simulink model "asbCubeSatVisualization"  (R2022a)
settings: configuration reference "CubeSatConfigSet" (kept outside this file)
undefined symbols (not defined in the file): altitude
libraries: aerolibutil x7, aerolibconvert2 x3, aerolibobsolete x1, aerolibattitudesys x1, simulink x1, vrlib x1
settings Model: DataDictionary=asbCubeSatArchInterfaceData.sldd  Creator=The MathWorks, Inc.  LastModifiedBy=4jack
settings ConfigSetRef: SourceName=CubeSatConfigSet

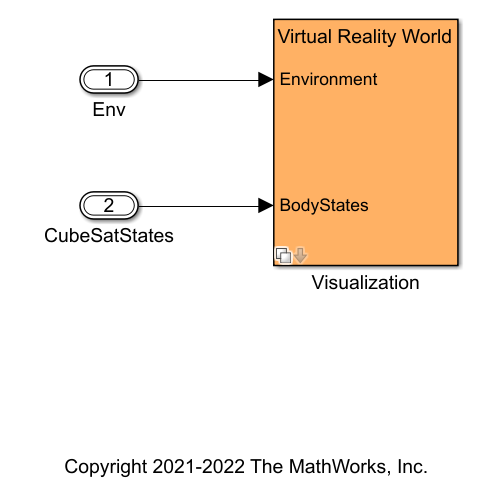
[thumbnail: Simulink's stored preview of the top-level diagram]
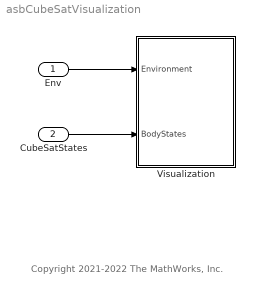
== system asbCubeSatVisualization ==
  note: Copyright 2021-2022 The MathWorks, Inc.
  Env : Inport  OutDataTypeStr=Bus: EnvBus
  CubeSatStates : Inport  Port=2  OutDataTypeStr=Bus: StatesOutBus
  Visualization : Subsystem  Variant=on  mask(Set Animation Properties){visSampleTime=5, cubesatSize=2e5, showAntenna=on, antennaHeight=-1*(altitude - 6317000), antennaHalfAngle=25}
      mask prompts: visSampleTime "spacecraft:cubesat:AnimSampleTime"; cubesatSize "spacecraft:cubesat:MdlSize"; showAntenna "spacecraft:cubesat:ShowCone"; antennaHeight "spacecraft:cubesat:ConeHeight"; antennaHalfAngle "spacecraft:cubesat:ConeAngle"
      mask help: spacecraft:cubesat:VisBlockDesc
      mask Callback showAntenna:
      | if builtin('license','test','Virtual_Reality_Toolbox')
      | 
      |     enable = get_param(gcb,'MaskEnables');
      |     if strcmp(get_param(gcb, 'showAntenna'), 'off')
      |         enable(4:5) = {'off'};
      |     else
      |         enable(4:5) = {'on'};
      |     end
      |     set_param(gcb,'MaskEnables', enable);
      |     clear enable
      | end
      mask DialogControl vrOpenBtn Prompt: spacecraft:cubesat:AnimOpenBtn
      mask DialogControl vrOpenBtn Callback:
      | if builtin('license','checkout','Virtual_Reality_Toolbox')
      |     vrmfunc('FnOpen',getSimulinkBlockHandle([gcb '/Virtual Reality World/VR Sink']));
      | end
      mask DialogControl visSampleTime Prompt: Animation refresh rate:
      mask DialogControl visSampleTime Tooltip: spacecraft:cubesat:AnimSampleTimeTT
      mask DialogControl cubesatSize Prompt: CubeSat display size [m]:
      mask DialogControl cubesatSize Tooltip: spacecraft:cubesat:MdlSizeTT
      mask DialogControl Container3 Prompt: spacecraft:cubesat:AntennaPropArea
      mask DialogControl showAntenna Prompt: Show antenna cone in animation
      mask DialogControl showAntenna Tooltip: spacecraft:cubesat:ShowConeTT
      mask DialogControl antennaHeight Prompt: Antenna cone height [m]:
      mask DialogControl antennaHeight Tooltip: spacecraft:cubesat:ConeHeightTT
      mask DialogControl antennaHalfAngle Prompt: Antenna cone half angle [deg]:
      mask DialogControl antennaHalfAngle Tooltip: spacecraft:cubesat:ConeAngleTT
  wires:
  CubeSatStates/1 -> Visualization/2(BodyStates)
  Env/1 -> Visualization/1(Environment)

== system asbCubeSatVisualization/Visualization ==
  Environment : Inport
  BodyStates : Inport  RequirementInfo={} %GIDa_10e629f3_1d72_465b_94cc_14990dd9aecc  Port=2
  No Visualization : Subsystem  VariantControl=visOff
  Virtual Reality World : Subsystem  VariantControl=visSL3D

== system asbCubeSatVisualization/Visualization/No Visualization ==
  BodyStates : Inport
  Environment : Inport  Port=2
  Terminator2 : Terminator
      settings: RequirementInfo={} %GIDa_0fc65eef_4c11_4565_975b_7fa0252905f4
  Terminator3 : Terminator
      settings: RequirementInfo={} %GIDa_377e63f1_3103_416f_a52c_127c2ec39819
  wires:
  BodyStates/1 -> Terminator3/1
  Environment/1 -> Terminator2/1

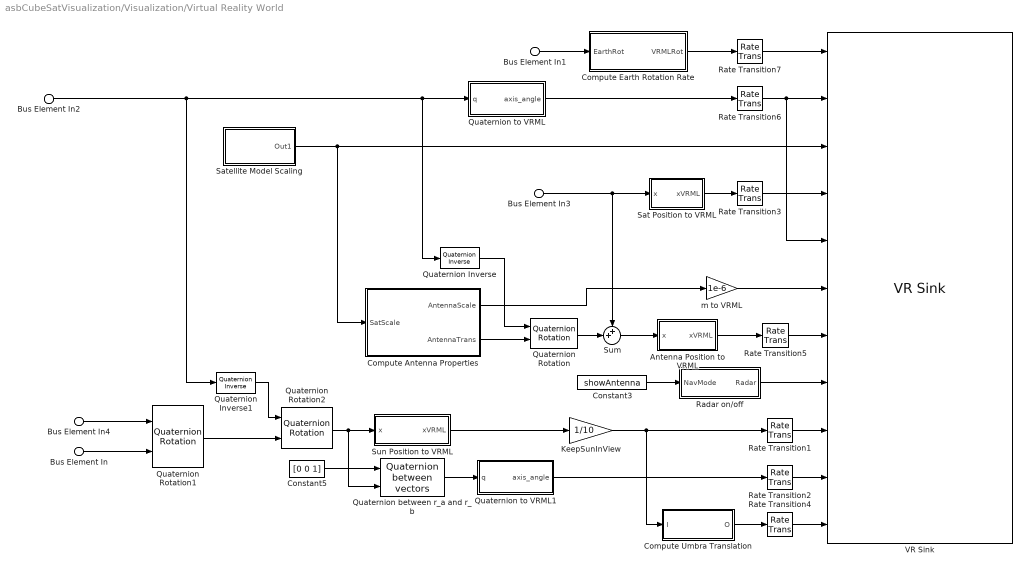
== system asbCubeSatVisualization/Visualization/Virtual Reality World ==
  Bus Element In3 : Inport  PortName=BodyStates  Element=X_ecef
  Bus Element In2 : Inport  PortName=BodyStates  Element=q_ecef2b
  Bus Element In4 : Inport  PortName=BodyStates  Element=q_eci2b
  Bus Element In : Inport  Port=2  PortName=Environment  Element=x_sun_eci
  Bus Element In1 : Inport  Port=2  PortName=Environment  Element=earthAngRate
  Antenna Position to VRML : Subsystem
  Compute Antenna Properties : Subsystem
  Compute Earth Rotation Rate : Subsystem
  Compute Umbra Translation : Subsystem
  Constant3 : Constant  Value=showAntenna
  Constant5 : Constant  Value=[0 0 1]
  KeepSunInView : Gain  Gain=1/10
  Quaternion Inverse : aerolibutil/Quaternion Inverse
  Quaternion Inverse1 : aerolibutil/Quaternion Inverse
  Quaternion Rotation : aerolibutil/Quaternion Rotation
  Quaternion Rotation1 : aerolibutil/Quaternion Rotation
  Quaternion Rotation2 : aerolibutil/Quaternion Rotation
  Quaternion between r_a and r_b : aerolibattitudesys/Quaternion between vectors
      settings: SourceProductBaseCode=AE
  Quaternion to VRML : Subsystem
  Quaternion to VRML1 : Subsystem
  Radar on/off : Subsystem
  Rate Transition{1..7} (7 alike) : RateTransition
  Sat Position to VRML : Subsystem
  Satellite Model Scaling : Subsystem
  Sum : Sum  Inputs=++|
  Sun Position to VRML : Subsystem
  VR Sink : vrlib/VR Sink  InstantiateOnLoad=on  SampleTime=visSampleTime  ViewEnable=on  RemoteChange=off  RemoteView=off  FieldsWritten=Earth.rotation.4.1.1.double#Satellite.rotation.4.1.1.double#Satellite.scale.3.1.1.double#Satellite.translation.3.1.1.double#AntennaCone.rotation.4.1.1.double#AntennaCone.scale.3.1.1.double#AntennaCone.translation.3.1.1.double#AntennaMaterial.transparency.1.1.1.double#Sun.translation.3.1.1.double#Umbra.rotation.4.1.1.double#Umbra.translation.3.1.1.double  WorldFileName=cubesatAnim.wrl  WorldDescription=CubeSat Orbit Animation  AutoView=on  VideoDimensions=[]  AllowVariableSize=off  FigureProperties="{'Position', 'Name', 'Viewpoint', 'CameraBound', 'CameraDirection', 'CameraPosition', 'CameraUpVector', 'ZoomFactor', 'Antialiasing', 'Headlight', 'Lighting', 'NavPanel', 'Sound', 'StatusBar', 'Stereo3D', 'Stereo3DCameraOffset', 'Stereo3DHIT', 'ToolBar', 'Textures', 'Transparency', 'Triad', 'Wireframe', 'NavZones', 'NavMode', 'NavSpeed', 'CaptureFileFormat', 'CaptureFileName', 'Record2DCompressMethod', 'Record2DCompressQuality', 'Record2D', 'Record2DFileName', 'Record2DFPS'; [5.0000000000000000e+00   9.2000000000000000e+01   5.7600000000000000e+02   3.5000000000000000e+02], 'CubeSat Orbit Animation', 'NorthPole', 'on', [0.0000000000000000e+00   0.0000000000000000e+00  -1.0000000000000000e+00], [0.0000000000000000e+00   0.0000000000000000e+00   0.0000000000000000e+00], [0.0000000000000000e+00   1.0000000000000000e+00   0.0000000000000000e+00], [1.0000000000000000e+00], 'on', 'on', 'on', 'halfbar', 'on', 'on', 'off', [1.0000000149011612e-01], [0.0000000000000000e+00], 'on', 'on', 'on', 'none', 'off', 'off', 'examine', 'normal', 'tif', '%f_anim_%n.tif', 'auto', [7.5000000000000000e+01], 'off', '%f_anim_%n.avi', 'auto'; [5.0000000000000000e+00   9.2000000000000000e+01   5.7600000000000000e+02   3.5000000000000000e+02], 'CubeSat Orbit Animation', 'NorthPole', 'on', [0.0000000000000000e+00   0.0000000000000000e+00  -1.0000000000000000e+00], [0.0000000000000000e+00   0.0000000000000000e+00   0.0000000000000000e+00], [0.0000000000000000e+00   1.0000000000000000e+00   0.0000000000000000e+00], [1.0000000000000000e+00], 'on', 'on', 'on', 'halfbar', 'on', 'on', 'off', [1.0000000149011612e-01], [0.0000000000000000e+00], 'on', 'on', 'on', 'none', 'off', 'off', 'examine', 'normal', 'tif', '%f_anim_%n.tif', 'auto', [7.5000000000000000e+01], 'off', '%f_anim_%n.avi', 'auto'}"
  m to VRML : Gain  Gain=1e-6
  wires:
  Rate Transition6/1 -> VR Sink/2, VR Sink/5
  Quaternion to VRML/1(axis_angle) -> Rate Transition6/1
  Rate Transition5/1 -> VR Sink/7
  Rate Transition3/1 -> VR Sink/4
  Rate Transition7/1 -> VR Sink/1
  Bus Element In1/1 -> Compute Earth Rotation Rate/1(EarthRot)
  Rate Transition2/1 -> VR Sink/10
  Rate Transition1/1 -> VR Sink/9
  Rate Transition4/1 -> VR Sink/11
  Bus Element In/1 -> Quaternion Rotation1/2
  Bus Element In4/1 -> Quaternion Rotation1/1
  Compute Antenna Properties/2(AntennaTrans) -> Quaternion Rotation/2
  Compute Antenna Properties/1(AntennaScale) -> m to VRML/1
  Satellite Model Scaling/1(Out1) -> Compute Antenna Properties/1(SatScale), VR Sink/3
  Compute Umbra Translation/1(O) -> Rate Transition4/1
  KeepSunInView/1 -> Rate Transition1/1, Compute Umbra Translation/1(I)
  Quaternion to VRML1/1(axis_angle) -> Rate Transition2/1
  Radar on/off/1(Radar) -> VR Sink/8
  Sat Position to VRML/1(xVRML) -> Rate Transition3/1
  Compute Earth Rotation Rate/1(VRMLRot) -> Rate Transition7/1
  Antenna Position to VRML/1(xVRML) -> Rate Transition5/1
  m to VRML/1 -> VR Sink/6
  Constant5/1 -> Quaternion between r_a and r_b/1
  Quaternion between r_a and r_b/1 -> Quaternion to VRML1/1(q)
  Sun Position to VRML/1(xVRML) -> KeepSunInView/1
  Quaternion Inverse1/1 -> Quaternion Rotation2/1
  Quaternion Rotation1/1 -> Quaternion Rotation2/2
  Quaternion Rotation2/1 -> Quaternion between r_a and r_b/2, Sun Position to VRML/1(x)
  Quaternion Rotation/1 -> Sum/2
  Sum/1 -> Antenna Position to VRML/1(x)
  Quaternion Inverse/1 -> Quaternion Rotation/1
  Bus Element In3/1 -> Sum/1, Sat Position to VRML/1(x)
  Constant3/1 -> Radar on/off/1(NavMode)
  Bus Element In2/1 -> Quaternion Inverse1/1, Quaternion Inverse/1, Quaternion to VRML/1(q)

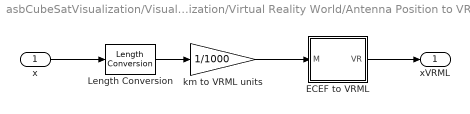
== system asbCubeSatVisualization/Visualization/Virtual Reality World/Antenna Position to VRML ==
  x : Inport
  ECEF to VRML : Subsystem
  Length Conversion : aerolibconvert2/Length Conversion  IU=m  OU=km
  km to VRML units : Gain  Gain=1/1000
  xVRML : Outport  VectorParamsAs1DForOutWhenUnconnected=off
  wires:
  ECEF to VRML/1(VR) -> xVRML/1
  x/1 -> Length Conversion/1
  km to VRML units/1 -> ECEF to VRML/1(M)
  Length Conversion/1 -> km to VRML units/1

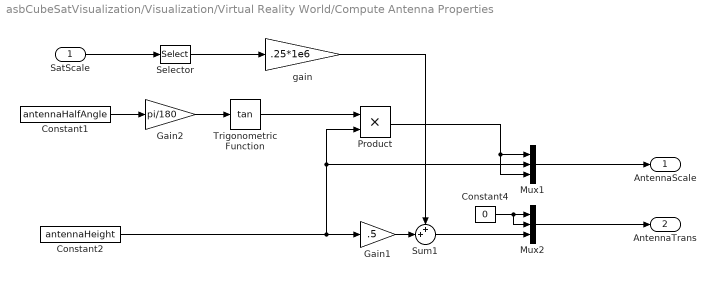
== system asbCubeSatVisualization/Visualization/Virtual Reality World/Compute Antenna Properties ==
  SatScale : Inport
  Constant1 : Constant  Value=antennaHalfAngle
  Constant2 : Constant  Value=antennaHeight
  Constant4 : Constant  Value=0
  Gain1 : Gain  Gain=.5
  Gain2 : Gain  Gain=pi/180
  Mux1 : Mux  Inputs=3
  Mux2 : Mux  Inputs=3
  Product : Product
  Selector : Selector  InputPortWidth=3  IndexOptions=Index vector (dialog)  Indices=1  OutputSizes=1
  Sum1 : Sum  Inputs=++|
  Trigonometric Function : Trigonometry  Operator=tan
  gain : Gain  Gain=.25*1e6
  AntennaScale : Outport  VectorParamsAs1DForOutWhenUnconnected=off
  AntennaTrans : Outport  Port=2  VectorParamsAs1DForOutWhenUnconnected=off
  wires:
  Selector/1 -> gain/1
  SatScale/1 -> Selector/1
  Mux1/1 -> AntennaScale/1
  Mux2/1 -> AntennaTrans/1
  Trigonometric Function/1 -> Product/1
  Gain1/1 -> Sum1/2
  Product/1 -> Mux1/1, Mux1/3
  Constant1/1 -> Gain2/1
  gain/1 -> Sum1/1
  Constant2/1 -> Product/2, Mux1/2, Gain1/1
  Sum1/1 -> Mux2/3
  Constant4/1 -> Mux2/2, Mux2/1
  Gain2/1 -> Trigonometric Function/1

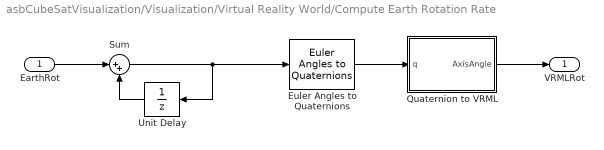
== system asbCubeSatVisualization/Visualization/Virtual Reality World/Compute Earth Rotation Rate ==
  EarthRot : Inport
  Euler Angles to Quaternions : aerolibobsolete/Euler Angles to Quaternions
      settings: SourceProductBaseCode=AE
  Quaternion to VRML : Subsystem
  Sum : Sum  Inputs=|++
  Unit Delay : UnitDelay  SampleTime=-1  HasFrameUpgradeWarning=on
  VRMLRot : Outport  VectorParamsAs1DForOutWhenUnconnected=off
  wires:
  Quaternion to VRML/1(AxisAngle) -> VRMLRot/1
  Euler Angles to Quaternions/1 -> Quaternion to VRML/1(q)
  Sum/1 -> Euler Angles to Quaternions/1, Unit Delay/1
  Unit Delay/1 -> Sum/2
  EarthRot/1 -> Sum/1

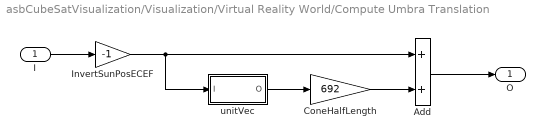
== system asbCubeSatVisualization/Visualization/Virtual Reality World/Compute Umbra Translation ==
  I : Inport
  Add : Sum
  ConeHalfLength : Gain  Gain=692
  InvertSunPosECEF : Gain  Gain=-1
  unitVec : Subsystem
  O : Outport  VectorParamsAs1DForOutWhenUnconnected=off
  wires:
  unitVec/1(O) -> ConeHalfLength/1
  InvertSunPosECEF/1 -> Add/1, unitVec/1(I)
  Add/1 -> O/1
  I/1 -> InvertSunPosECEF/1
  ConeHalfLength/1 -> Add/2

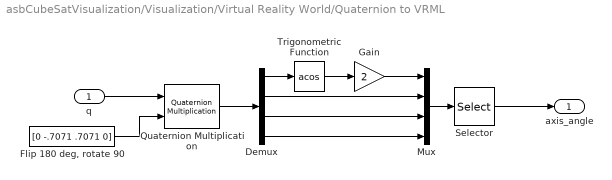
== system asbCubeSatVisualization/Visualization/Virtual Reality World/Quaternion to VRML ==
  q : Inport
  Demux : Demux
  "Flip 180 deg, rotate 90" : Constant  Value=[0 -.7071 .7071 0]
  Gain : Gain  Gain=2
  Mux : Mux
  Quaternion Multiplication : aerolibutil/Quaternion Multiplication
  Selector : Selector  InputPortWidth=4  IndexOptions=Index vector (dialog)  Indices=[3 4 2 1]  OutputSizes=1
  Trigonometric Function : Trigonometry  Operator=acos
  axis_angle : Outport  VectorParamsAs1DForOutWhenUnconnected=off
  wires:
  Quaternion Multiplication/1 -> Demux/1
  "Flip 180 deg, rotate 90"/1 -> Quaternion Multiplication/2
  Demux/1 -> Trigonometric Function/1
  Trigonometric Function/1 -> Gain/1
  Mux/1 -> Selector/1
  q/1 -> Quaternion Multiplication/1
  Selector/1 -> axis_angle/1
  Gain/1 -> Mux/1
  Demux/2 -> Mux/2
  Demux/3 -> Mux/3
  Demux/4 -> Mux/4

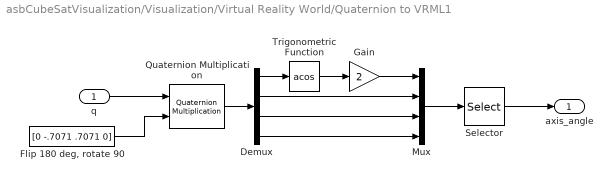
== system asbCubeSatVisualization/Visualization/Virtual Reality World/Quaternion to VRML1 ==
  q : Inport
  Demux : Demux
  "Flip 180 deg, rotate 90" : Constant  Value=[0 -.7071 .7071 0]
  Gain : Gain  Gain=2
  Mux : Mux
  Quaternion Multiplication : aerolibutil/Quaternion Multiplication
  Selector : Selector  InputPortWidth=4  IndexOptions=Index vector (dialog)  Indices=[3 4 2 1]  OutputSizes=1
  Trigonometric Function : Trigonometry  Operator=acos
  axis_angle : Outport  VectorParamsAs1DForOutWhenUnconnected=off
  wires:
  Quaternion Multiplication/1 -> Demux/1
  q/1 -> Quaternion Multiplication/1
  "Flip 180 deg, rotate 90"/1 -> Quaternion Multiplication/2
  Demux/1 -> Trigonometric Function/1
  Trigonometric Function/1 -> Gain/1
  Mux/1 -> Selector/1
  Selector/1 -> axis_angle/1
  Gain/1 -> Mux/1
  Demux/2 -> Mux/2
  Demux/3 -> Mux/3
  Demux/4 -> Mux/4

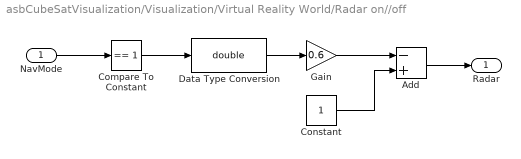
== system asbCubeSatVisualization/Visualization/Virtual Reality World/Radar on//off ==
  NavMode : Inport
  Add : Sum  Inputs=-+
  Compare To Constant : simulink/Logic and Bit Operations/Compare To Constant  relop===  const=1  OutDataTypeStr=boolean  ZeroCross=off
  Constant : Constant
  Data Type Conversion : DataTypeConversion  OutDataTypeStr=double  SaturateOnIntegerOverflow=off  RndMeth=Floor
  Gain : Gain  Gain=0.6
  Radar : Outport  VectorParamsAs1DForOutWhenUnconnected=off
  wires:
  Add/1 -> Radar/1
  Constant/1 -> Add/2
  Gain/1 -> Add/1
  Data Type Conversion/1 -> Gain/1
  Compare To Constant/1 -> Data Type Conversion/1
  NavMode/1 -> Compare To Constant/1

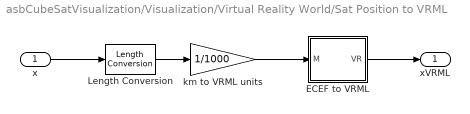
== system asbCubeSatVisualization/Visualization/Virtual Reality World/Sat Position to VRML ==
  x : Inport
  ECEF to VRML : Subsystem
  Length Conversion : aerolibconvert2/Length Conversion  IU=m  OU=km
  km to VRML units : Gain  Gain=1/1000
  xVRML : Outport  VectorParamsAs1DForOutWhenUnconnected=off
  wires:
  Length Conversion/1 -> km to VRML units/1
  km to VRML units/1 -> ECEF to VRML/1(M)
  x/1 -> Length Conversion/1
  ECEF to VRML/1(VR) -> xVRML/1

== system asbCubeSatVisualization/Visualization/Virtual Reality World/Satellite Model Scaling ==
  Constant : Constant  Value=cubesatSize
  Mux : Mux  Inputs=3
  ScaleModelToVRML : Gain  Gain=1/.3e6
  Out1 : Outport  VectorParamsAs1DForOutWhenUnconnected=off
  wires:
  Mux/1 -> Out1/1
  Constant/1 -> ScaleModelToVRML/1
  ScaleModelToVRML/1 -> Mux/2, Mux/1, Mux/3

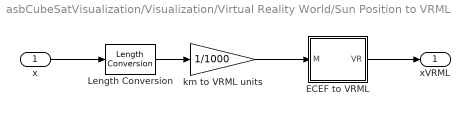
== system asbCubeSatVisualization/Visualization/Virtual Reality World/Sun Position to VRML ==
  x : Inport
  ECEF to VRML : Subsystem
  Length Conversion : aerolibconvert2/Length Conversion  IU=m  OU=km
  km to VRML units : Gain  Gain=1/1000
  xVRML : Outport  VectorParamsAs1DForOutWhenUnconnected=off
  wires:
  Length Conversion/1 -> km to VRML units/1
  km to VRML units/1 -> ECEF to VRML/1(M)
  x/1 -> Length Conversion/1
  ECEF to VRML/1(VR) -> xVRML/1

== system asbCubeSatVisualization/Visualization/Virtual Reality World/Antenna Position to VRML/ECEF to VRML ==
  M : Inport  PortDimensions=3
  Selector : Selector  InputPortWidth=3  IndexOptions=Index vector (dialog)  Indices=[2 3 1]  OutputSizes=1
  VR : Outport  PortDimensions=3  VectorParamsAs1DForOutWhenUnconnected=off
  wires:
  Selector/1 -> VR/1
  M/1 -> Selector/1

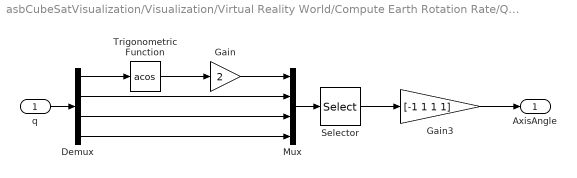
== system asbCubeSatVisualization/Visualization/Virtual Reality World/Compute Earth Rotation Rate/Quaternion to VRML ==
  q : Inport
  Demux : Demux
  Gain : Gain  Gain=2
  Gain3 : Gain  Gain=[-1 1 1 1]
  Mux : Mux
  Selector : Selector  InputPortWidth=4  IndexOptions=Index vector (dialog)  Indices=[2 4 3 1]  OutputSizes=1
  Trigonometric Function : Trigonometry  Operator=acos
  AxisAngle : Outport  VectorParamsAs1DForOutWhenUnconnected=off
  wires:
  Demux/1 -> Trigonometric Function/1
  Trigonometric Function/1 -> Gain/1
  Mux/1 -> Selector/1
  q/1 -> Demux/1
  Gain3/1 -> AxisAngle/1
  Selector/1 -> Gain3/1
  Gain/1 -> Mux/1
  Demux/2 -> Mux/2
  Demux/3 -> Mux/3
  Demux/4 -> Mux/4

== system asbCubeSatVisualization/Visualization/Virtual Reality World/Compute Umbra Translation/unitVec ==
  I : Inport
  Divide : Product  Inputs=*/
  Dot Product : DotProduct  OutDataTypeStr=Inherit: Inherit via internal rule
  Sqrt : Sqrt
  O : Outport  VectorParamsAs1DForOutWhenUnconnected=off
  wires:
  Sqrt/1 -> Divide/2
  Divide/1 -> O/1
  I/1 -> Dot Product/2, Dot Product/1, Divide/1
  Dot Product/1 -> Sqrt/1

== system asbCubeSatVisualization/Visualization/Virtual Reality World/Sat Position to VRML/ECEF to VRML ==
  M : Inport  PortDimensions=3
  Selector : Selector  InputPortWidth=3  IndexOptions=Index vector (dialog)  Indices=[2 3 1]  OutputSizes=1
  VR : Outport  PortDimensions=3  VectorParamsAs1DForOutWhenUnconnected=off
  wires:
  Selector/1 -> VR/1
  M/1 -> Selector/1

== system asbCubeSatVisualization/Visualization/Virtual Reality World/Sun Position to VRML/ECEF to VRML ==
  M : Inport  PortDimensions=3
  Selector : Selector  InputPortWidth=3  IndexOptions=Index vector (dialog)  Indices=[2 3 1]  OutputSizes=1
  VR : Outport  PortDimensions=3  VectorParamsAs1DForOutWhenUnconnected=off
  wires:
  Selector/1 -> VR/1
  M/1 -> Selector/1
